simulink model "WECS_QuadraticBoost_Circuit_v2"  (R2024a)
settings: Solver=ode23tb  StartTime=0.0  StopTime=50.0  MaxStep=1e-5  RelTol=1e-3
libraries: spsSeriesRLCBranchLib x6, spsDiodeLib x3, spsGroundLib x2, spsCurrentMeasurementLib x2, spsVoltageMeasurementLib x2, spsDCVoltageSourceLib x1, simulink x1, spsMosfetLib x1, spspowerguiLib x1
settings Model: Creator=saranboddu  LastModifiedBy=saranboddu

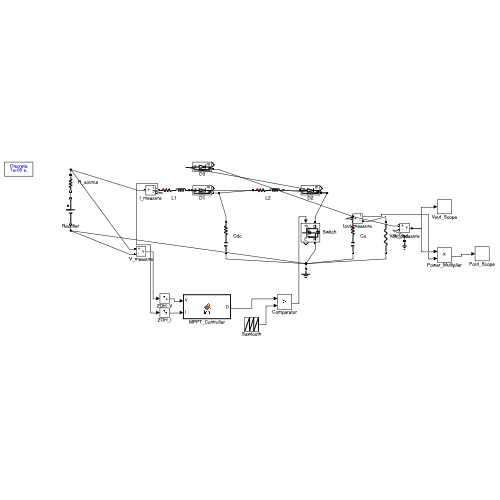
[thumbnail: Simulink's stored preview of the top-level diagram]
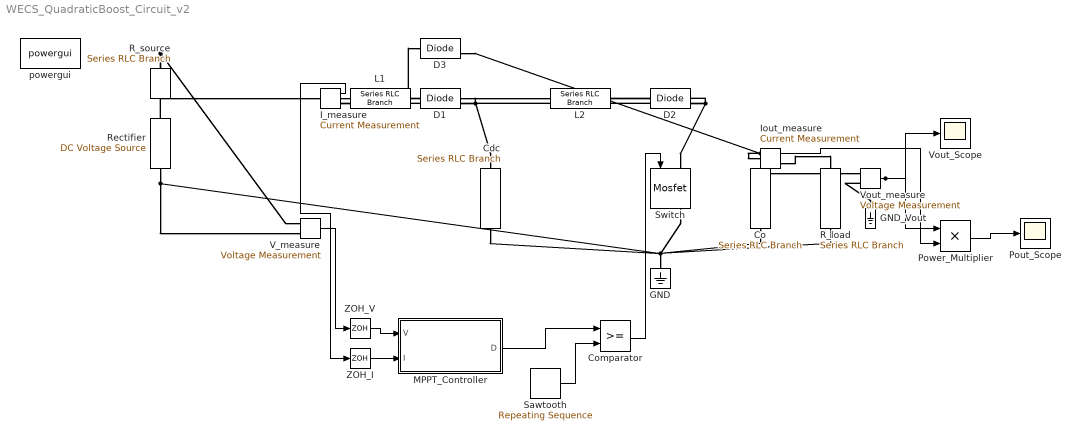
== system WECS_QuadraticBoost_Circuit_v2 ==
  Cdc : spsSeriesRLCBranchLib/Series RLC Branch  LConnTagsString=__new0  RConnTagsString=__new0  BranchType=RC  Resistance=0.01  Inductance=1e-3  SetiL0=off  InitialCurrent=0  Capacitance=3.1e-07  Setx0=off  InitialVoltage=0  Measurements=None
  Co : spsSeriesRLCBranchLib/Series RLC Branch  LConnTagsString=__new0  RConnTagsString=__new0  BranchType=RC  Resistance=0.01  Inductance=1e-3  SetiL0=off  InitialCurrent=0  Capacitance=1.9e-07  Setx0=off  InitialVoltage=0  Measurements=None
  Comparator : RelationalOperator  OutDataTypeStr=boolean  RndMeth=Simplest  InputSameDT=off
  D1 : spsDiodeLib/Diode  Ron=0.001  Lon=0  Vf=0.8  IC=0  UseSnubber=0  Rs=500  Cs=250e-9  Measurements=on
  D2 : spsDiodeLib/Diode  Ron=0.001  Lon=0  Vf=0.8  IC=0  UseSnubber=0  Rs=500  Cs=250e-9  Measurements=on
  D3 : spsDiodeLib/Diode  Ron=0.001  Lon=0  Vf=0.8  IC=0  UseSnubber=0  Rs=500  Cs=250e-9  Measurements=on
  GND : spsGroundLib/Ground  LConnTagsString=a
  GND_Vout : spsGroundLib/Ground  LConnTagsString=a
  I_measure : spsCurrentMeasurementLib/Current Measurement  PhasorSimulation=off  OutputType=Complex  PSBequivalent=0
  Iout_measure : spsCurrentMeasurementLib/Current Measurement  PhasorSimulation=off  OutputType=Complex  PSBequivalent=0
  L1 : spsSeriesRLCBranchLib/Series RLC Branch  LConnTagsString=__new0  RConnTagsString=__new0  BranchType=RL  Resistance=0.1  Inductance=7.73e-05  SetiL0=off  InitialCurrent=0  Capacitance=1e-6  Setx0=off  InitialVoltage=0  Measurements=None
  L2 : spsSeriesRLCBranchLib/Series RLC Branch  LConnTagsString=__new0  RConnTagsString=__new0  BranchType=RL  Resistance=0.1  Inductance=9.973e-05  SetiL0=off  InitialCurrent=0  Capacitance=1e-6  Setx0=off  InitialVoltage=0  Measurements=None
  MPPT_Controller : MATLAB Function  TreatAsAtomicUnit=on
  Pout_Scope : Scope
  Power_Multiplier : Product
  R_load : spsSeriesRLCBranchLib/Series RLC Branch  LConnTagsString=__new0  RConnTagsString=__new0  BranchType=R  Resistance=48.13  Inductance=1e-3  SetiL0=off  InitialCurrent=0  Capacitance=1e-6  Setx0=off  InitialVoltage=0  Measurements=None
  R_source : spsSeriesRLCBranchLib/Series RLC Branch  LConnTagsString=__new0  RConnTagsString=__new0  BranchType=R  Resistance=5  Inductance=1e-3  SetiL0=off  InitialCurrent=0  Capacitance=1e-6  Setx0=off  InitialVoltage=0  Measurements=None
  Rectifier : spsDCVoltageSourceLib/DC Voltage Source  Amplitude=540  Measurements=None
  Sawtooth : simulink/Sources/Repeating Sequence  rep_seq_t=[0 1/24000]  rep_seq_y=[0 1]
  Switch : spsMosfetLib/Mosfet  Ron=0.1  Lon=0  Rd=0.01  Vfd=0  IC=0  Rs=1e5  Cs=inf  Measurements=on
  V_measure : spsVoltageMeasurementLib/Voltage Measurement  PhasorSimulation=off  OutputType=Complex  PSBequivalent=0
  Vout_Scope : Scope
  Vout_measure : spsVoltageMeasurementLib/Voltage Measurement  PhasorSimulation=off  OutputType=Complex  PSBequivalent=0
  ZOH_I : ZeroOrderHold  SampleTime=-1
  ZOH_V : ZeroOrderHold  SampleTime=-1
  powergui : spspowerguiLib/powergui  Priority=1  SimulationMode=Discrete  SampleTime=10e-6  frequency=60  Iterations=50  frequencyindice=60  Pbase=100e6  ErrMax=1e-4  UnitsV=kV  UnitsW=MW  buscounter=0  FunctionMessages=off  echomessages=off  EnableUseOfTLC=off  CurrentSourceSwitches=off  DisableSnubberDevices=off  DisableRonSwitches=off  DisableVfSwitches=off  DisplayEquations=off  AutomaticDiscreteSolvers=off  SolverType=Tustin/Backward Euler (TBE)  Interpol=off  ExternalGateDelay=off  methode=off  Ts=100  x0status=blocks  SPID=on  SwTol=0  HookPort=off  NonlinearTolerance=1e-4  nMaxIteration=100  ContinueOnMaxIteration=off  RestoreLinks=warning  ResistiveCurrentMeasurement=off  Frange=[0:2:500]  Ylog=off  Xlog=on  ShowGrid=off  save=off  variable=ZData  structure=0  ZoomFFT=off  StartTime=0.0  cycles=1  DisplayStyle=1  fundamental=60  FreqAxis=off  MaxFrequency=1000  frequencyindicesteady=1  RmsSteady=1  display=off
  wires:
  V_measure/1 -> ZOH_V/1
  I_measure/1 -> ZOH_I/1
  ZOH_V/1 -> MPPT_Controller/1(V)
  ZOH_I/1 -> MPPT_Controller/2(I)
  MPPT_Controller/1(D) -> Comparator/1
  Sawtooth/1 -> Comparator/2
  Comparator/1 -> Switch/1
  Vout_measure/1 -> Vout_Scope/1, Power_Multiplier/1
  Iout_measure/1 -> Power_Multiplier/2
  Power_Multiplier/1 -> Pout_Scope/1
  connections:
  Rectifier/LConn1 -- V_measure/LConn2 -- Cdc/RConn1 -- Co/RConn1 -- R_load/RConn1 -- GND/LConn1 -- Switch/RConn1
  D1/LConn1 -- L1/RConn1 -- D2/LConn1
  Cdc/LConn1 -- D1/RConn1 -- L2/LConn1
  Switch/LConn1 -- D2/RConn1 -- L2/RConn1 -- D3/LConn1
  D3/RConn1 -- Iout_measure/LConn1 -- Co/LConn1 -- Vout_measure/LConn1
  Rectifier/RConn1 -- R_source/LConn1
  V_measure/LConn1 -- R_source/RConn1 -- I_measure/LConn1
  I_measure/RConn1 -- L1/LConn1
  Iout_measure/RConn1 -- R_load/LConn1
  Vout_measure/LConn2 -- GND_Vout/LConn1

== matlab function WECS_QuadraticBoost_Circuit_v2/MPPT_Controller ==
  data: V input; D output; I input
function D = MPPT_Flowchart(V, I)
% MPPT_Flowchart implements the Incremental Conductance algorithm
% based on the flowchart in Figure 3 of the reference paper.

    % Persistent variables to store previous state
    persistent V_prev I_prev D_prev;
    
    if isempty(V_prev)
        V_prev = 0;
        I_prev = 0;
        D_prev = 0.5; % Initial duty cycle
    end
    
    % Calculate variations
    dV = V - V_prev;
    dI = I - I_prev;
    
    % Step size
    step = 0.002;
    
    if abs(dV) < 0.1 % dV == 0 condition
        if dI > 0.05 % dI > 0 condition
            % Increase V_ref means decrease Duty cycle in Boost converters
            D_prev = D_prev - step;
        elseif dI < -0.05
            % Decrease V_ref means increase Duty cycle
            D_prev = D_prev + step;
        end
    else
        % dV ~= 0
        % Incremental conductance condition: dI/dV == -I/V  => dI*V + dV*I == 0
        inc_cond = dI/dV + I/V;
        
        if abs(inc_cond) > 0.01 % Not optimal
            if inc_cond > 0
                % dI/dV > -I/V -> Increase V_ref -> Decrease Duty Cycle
                D_prev = D_prev - step;
            else
                % Decrease V_ref -> Increase Duty Cycle
                D_prev = D_prev + step;
            end
        end
    end
    
    % Bound Duty Cycle
    if D_prev > 0.5
        D_prev = 0.9;
    elseif D_prev < 0.1
        D_prev = 0.1;
    end
    
    D = D_prev;
    
    % Update previous values
    V_prev = V;
    I_prev = I;
end
